simulink model "Import_IMU"  (R2023b)
settings: Solver=FixedStepDiscrete  StartTime=0.0  StopTime=inf  FixedStep=0.003  RelTol=1e-3
InitFcn:
  | run('dual_leg_init.m');
values from neighbouring files (symbols this model uses):
  L1 = single(0.0804)    [dual_leg_init.m]
  L2 = single(0.1200)    [dual_leg_init.m]
  L3 = single(0.1200)    [dual_leg_init.m]
  L4 = single(0.0804)    [dual_leg_init.m]
  L5 = single(0.0700)    [dual_leg_init.m]
undefined symbols (not defined in the file or in its folder): CAL
libraries: ros2lib x14
(part 2 of 2)

== matlab function Import_IMU/FiveBar_IK_Right ==
  data: xCmd input; alphaCmd output; yCmd input; alphaActual input; betaActual input; L1 input; L2 input; L3 input; L4 input; L5 input; betaCmd output; valid output
function [alphaCmd, betaCmd, valid] = fivebar_ik( ...
    xCmd, yCmd, ...
    alphaActual, betaActual, ...
    L1, L2, L3, L4, L5)
%#codegen
%
% Five-Bar Inverse Kinematics
% 五连杆逆运动学
%
% 功能：
% 已知轮毂中心目标坐标(xCmd,yCmd)，
% 求两个主动关节目标角alphaCmd、betaCmd。
%
% 坐标定义：
%
% Alpha电机中心：
%   O = (0,0)
%
% Beta电机中心：
%   D = (L5,0)
%
% 腿部局部坐标：
%   +x：Alpha电机指向Beta电机
%   +y：竖直向下
%
% 连杆：
%   O-A = L1
%   A-B = L2
%   D-C = L4
%   C-B = L3
%
% 输入：
%   xCmd        轮毂目标x，单位m
%   yCmd        轮毂目标y，单位m
%   alphaActual 当前实际Alpha关节角，单位rad
%   betaActual  当前实际Beta关节角，单位rad
%   L1~L5       五连杆尺寸，单位m
%
% 输出：
%   alphaCmd    Alpha关节目标角，单位rad
%   betaCmd     Beta关节目标角，单位rad
%   valid       目标位置是否可达
%
% 解选择方法：
% 每个主动关节都会产生两个候选解，
% 本函数选择最接近当前实际关节角的解，
% 避免机构突然跳到另一种装配构型。

%% 默认输出

alphaCmd = alphaActual;
betaCmd  = betaActual;
valid    = false;

%% 检查输入是否有效

inputValid = ...
    isfinite(xCmd)        && ...
    isfinite(yCmd)        && ...
    isfinite(alphaActual) && ...
    isfinite(betaActual)  && ...
    isfinite(L1)          && ...
    isfinite(L2)          && ...
    isfinite(L3)          && ...
    isfinite(L4)          && ...
    isfinite(L5);

if ~inputValid
    return;
end

if L1 <= single(0) || ...
   L2 <= single(0) || ...
   L3 <= single(0) || ...
   L4 <= single(0) || ...
   L5 <= single(0)

    return;
end

%% =========================================================
%  求Alpha侧两个候选解
%
%  Alpha电机中心O = (0,0)
%  主动杆长度L1
%  被动杆长度L2
% ==========================================================

dxAlpha = xCmd;
dyAlpha = yCmd;

rAlphaSquared = ...
    dxAlpha * dxAlpha + ...
    dyAlpha * dyAlpha;

rAlpha = sqrt(rAlphaSquared);

% 检查目标是否在Alpha侧二连杆工作空间内
if rAlpha < single(1.0e-6)
    return;
end

if rAlpha > L1 + L2
    return;
end

if rAlpha < abs(L1 - L2)
    return;
end

% 从余弦定理求主动杆与目标连线之间的夹角
cosDeltaAlpha = ...
    (L1 * L1 + rAlphaSquared - L2 * L2) / ...
    (single(2) * L1 * rAlpha);

% 处理浮点数误差
tolerance = single(1.0e-5);

if cosDeltaAlpha > single(1) + tolerance || ...
   cosDeltaAlpha < single(-1) - tolerance

    return;
end

if cosDeltaAlpha > single(1)
    cosDeltaAlpha = single(1);
elseif cosDeltaAlpha < single(-1)
    cosDeltaAlpha = single(-1);
end

phiAlpha = atan2(dyAlpha, dxAlpha);
deltaAlpha = acos(cosDeltaAlpha);

% Alpha两个候选角
alphaCandidate1 = phiAlpha + deltaAlpha;
alphaCandidate2 = phiAlpha - deltaAlpha;

%% =========================================================
%  求Beta侧两个候选解
%
%  Beta电机中心D = (L5,0)
%  主动杆长度L4
%  被动杆长度L3
% ==========================================================

dxBeta = xCmd - L5;
dyBeta = yCmd;

rBetaSquared = ...
    dxBeta * dxBeta + ...
    dyBeta * dyBeta;

rBeta = sqrt(rBetaSquared);

% 检查目标是否在Beta侧二连杆工作空间内
if rBeta < single(1.0e-6)
    return;
end

if rBeta > L4 + L3
    return;
end

if rBeta < abs(L4 - L3)
    return;
end

cosDeltaBeta = ...
    (L4 * L4 + rBetaSquared - L3 * L3) / ...
    (single(2) * L4 * rBeta);

if cosDeltaBeta > single(1) + tolerance || ...
   cosDeltaBeta < single(-1) - tolerance

    return;
end

if cosDeltaBeta > single(1)
    cosDeltaBeta = single(1);
elseif cosDeltaBeta < single(-1)
    cosDeltaBeta = single(-1);
end

phiBeta = atan2(dyBeta, dxBeta);
deltaBeta = acos(cosDeltaBeta);

% Beta两个候选角
betaCandidate1 = phiBeta + deltaBeta;
betaCandidate2 = phiBeta - deltaBeta;

%% =========================================================
%  将候选角转换到当前实际关节角附近
%
%  例如：
%  当前角为3.2 rad，
%  候选角为-3.0 rad，
%  实际上二者可能只相差约0.08 rad。
% ==========================================================

alphaCandidate1 = alphaActual + ...
    wrap_to_pi_single(alphaCandidate1 - alphaActual);

alphaCandidate2 = alphaActual + ...
    wrap_to_pi_single(alphaCandidate2 - alphaActual);

betaCandidate1 = betaActual + ...
    wrap_to_pi_single(betaCandidate1 - betaActual);

betaCandidate2 = betaActual + ...
    wrap_to_pi_single(betaCandidate2 - betaActual);

%% 选择距离当前实际角最近的Alpha解

alphaError1 = abs(alphaCandidate1 - alphaActual);
alphaError2 = abs(alphaCandidate2 - alphaActual);

if alphaError1 <= alphaError2
    alphaCmd = alphaCandidate1;
else
    alphaCmd = alphaCandidate2;
end

%% 选择距离当前实际角最近的Beta解

betaError1 = abs(betaCandidate1 - betaActual);
betaError2 = abs(betaCandidate2 - betaActual);

if betaError1 <= betaError2
    betaCmd = betaCandidate1;
else
    betaCmd = betaCandidate2;
end

%% 最终有效性检查

if ~isfinite(alphaCmd) || ~isfinite(betaCmd)
    alphaCmd = alphaActual;
    betaCmd  = betaActual;
    return;
end

valid = true;

end


function angleWrapped = wrap_to_pi_single(angle)
% 将角度限制到[-pi,pi)

piSingle = single(pi);
twoPi = single(2) * piSingle;

angleWrapped = mod(angle + piSingle, twoPi) - piSingle;

end

== matlab function Import_IMU/Right_leg/Right_Joint_To_Motor_R ==
  data: alpha_cmd input; p_RA_target output; beta_cmd input; p_RB_target output; valid output
function [p_RA_target, p_RB_target, valid] = ...
    Right_Joint_To_Motor(alpha_cmd, beta_cmd)
%#codegen
% 将左腿两个主动关节目标角转换为电机目标角

% RA标定参数
qm0_RA   = single(-0.9126806259155273);
qj0_RA   = single(2.2416795698181398);
sign_RA  = single( 1.0);
ratio_RA = single( 1.0);

% RB标定参数
qm0_RB   = single(-0.6025409698486328);
qj0_RB   = single(-0.36295295726680576);
sign_RB  = single( 1.0);
ratio_RB = single( 1.0);

alpha_cmd = single(alpha_cmd);
beta_cmd  = single(beta_cmd);

p_RA_target = qm0_RA + ...
    (alpha_cmd - qj0_RA) * ratio_RA / sign_RA;

p_RB_target = qm0_RB + ...
    (beta_cmd - qj0_RB) * ratio_RB / sign_RB;

valid = ...
    isfinite(p_RA_target) && ...
    isfinite(p_RB_target);

end

== matlab function Import_IMU/Right_leg/Motor_Target_Velocity_LA ==
  data: p_cmd input; v_des output; enable input; Ts input; cutoff_hz input; max_velocity input; valid output
function [v_des, valid] = Motor_Target_Velocity( ...
    p_cmd, enable, Ts, cutoff_hz, max_velocity)
%#codegen
% 根据最终电机位置目标计算速度目标
%
% p_cmd        最终发送的电机目标位置，rad
% enable       控制使能
% Ts           控制周期，s
% cutoff_hz    速度低通滤波截止频率，Hz
% max_velocity 目标速度限制，rad/s

persistent p_previous
persistent v_previous
persistent was_enabled

if isempty(p_previous)
    p_previous = single(0);
    v_previous = single(0);
    was_enabled = false;
end

p_cmd        = single(p_cmd);
Ts           = single(Ts);
cutoff_hz    = single(cutoff_hz);
max_velocity = single(max_velocity);

v_des = single(0);
valid = false;

control_enabled = enable ~= 0;

if ~control_enabled
    p_previous = p_cmd;
    v_previous = single(0);
    was_enabled = false;
    return;
end

if ~isfinite(p_cmd) || ...
   ~isfinite(Ts) || ...
   ~isfinite(cutoff_hz) || ...
   ~isfinite(max_velocity)
    return;
end

if Ts <= single(1.0e-6)
    return;
end

% 刚使能时避免产生巨大差分速度
if ~was_enabled
    p_previous = p_cmd;
    v_previous = single(0);
    was_enabled = true;

    v_des = single(0);
    valid = true;
    return;
end

% 原始差分速度
v_raw = (p_cmd - p_previous) / Ts;

% 速度限幅
v_raw = min(max(v_raw, -max_velocity), max_velocity);

% 一阶低通滤波
if cutoff_hz > single(0)
    filter_coefficient = ...
        exp(-single(2.0*pi) * cutoff_hz * Ts);

    v_des = ...
        filter_coefficient * v_previous + ...
        (single(1.0) - filter_coefficient) * v_raw;
else
    v_des = v_raw;
end

% 再做一次限幅
v_des = min(max(v_des, -max_velocity), max_velocity);

p_previous = p_cmd;
v_previous = v_des;

valid = isfinite(v_des);

end

== matlab function Import_IMU/Right_leg/Motor_Target_Velocity_LB ==
  data: p_cmd input; v_des output; enable input; Ts input; cutoff_hz input; max_velocity input; valid output
function [v_des, valid] = Motor_Target_Velocity( ...
    p_cmd, enable, Ts, cutoff_hz, max_velocity)
%#codegen
% 根据最终电机位置目标计算速度目标
%
% p_cmd        最终发送的电机目标位置，rad
% enable       控制使能
% Ts           控制周期，s
% cutoff_hz    速度低通滤波截止频率，Hz
% max_velocity 目标速度限制，rad/s

persistent p_previous
persistent v_previous
persistent was_enabled

if isempty(p_previous)
    p_previous = single(0);
    v_previous = single(0);
    was_enabled = false;
end

p_cmd        = single(p_cmd);
Ts           = single(Ts);
cutoff_hz    = single(cutoff_hz);
max_velocity = single(max_velocity);

v_des = single(0);
valid = false;

control_enabled = enable ~= 0;

if ~control_enabled
    p_previous = p_cmd;
    v_previous = single(0);
    was_enabled = false;
    return;
end

if ~isfinite(p_cmd) || ...
   ~isfinite(Ts) || ...
   ~isfinite(cutoff_hz) || ...
   ~isfinite(max_velocity)
    return;
end

if Ts <= single(1.0e-6)
    return;
end

% 刚使能时避免产生巨大差分速度
if ~was_enabled
    p_previous = p_cmd;
    v_previous = single(0);
    was_enabled = true;

    v_des = single(0);
    valid = true;
    return;
end

% 原始差分速度
v_raw = (p_cmd - p_previous) / Ts;

% 速度限幅
v_raw = min(max(v_raw, -max_velocity), max_velocity);

% 一阶低通滤波
if cutoff_hz > single(0)
    filter_coefficient = ...
        exp(-single(2.0*pi) * cutoff_hz * Ts);

    v_des = ...
        filter_coefficient * v_previous + ...
        (single(1.0) - filter_coefficient) * v_raw;
else
    v_des = v_raw;
end

% 再做一次限幅
v_des = min(max(v_des, -max_velocity), max_velocity);

p_previous = p_cmd;
v_previous = v_des;

valid = isfinite(v_des);

end

== matlab function Import_IMU/Switch/RC_Safety_Gate ==
  data: isNew input; enable_safe output; online input; rightSwitch input; rc_alive output; rc_ready output; status output
function [enable_safe,rc_alive,rc_ready,status] = ...
    RC_Safety_Gate(isNew,online,rightSwitch)
%#codegen
%
% isNew       : ROS 2 Subscribe的IsNew端口，boolean
% online      : ReadDJIRC.online，uint8
% rightSwitch : ReadDJIRC.right_switch，uint8
%
% enable_safe : 最终安全使能
% rc_alive    : 遥控器通信正常
% rc_ready    : 已经先经过失能挡，可以允许使能
% status      : 状态码，方便调试

persistent missedCount receivedOnce seenDisable

if isempty(missedCount)
    % 启动时直接处于超时状态
    missedCount = uint32(34);
    receivedOnce = false;
    seenDisable = false;
end

% 当前模型Ts = 0.003 s
% 0.1 / 0.003 = 33.33
% 所以连续34个周期没有新消息就判定超时
TIMEOUT_STEPS = uint32(34);

%% 1. 新消息计数与超时判断
if isNew
    missedCount = uint32(0);
    receivedOnce = true;
else
    if missedCount < uint32(1000000)
        missedCount = missedCount + uint32(1);
    end
end

fresh = receivedOnce && ...
        (missedCount < TIMEOUT_STEPS);

%% 2. 检查遥控器消息是否合法
% 你的右侧三档开关正常值应为1、2、3
switchValid = ...
    (rightSwitch >= uint8(1)) && ...
    (rightSwitch <= uint8(3));

rc_alive = fresh && ...
           (online ~= uint8(0)) && ...
           switchValid;

%% 3. 启动互锁
% 一旦断线，清除“见过失能挡”的记录。
% 这样重新连接时，即使开关仍在3挡，也不会自动使能。
if ~rc_alive
    seenDisable = false;
else
    % 当前模型中 right_switch > 2 才使能，
    % 因此1挡和2挡都看作失能状态。
    if rightSwitch <= uint8(2)
        seenDisable = true;
    end
end

rc_ready = rc_alive && seenDisable;

%% 4. 最终使能
% 必须：
% 通信正常
% 已经先经过失能挡
% 当前开关位于3挡
enable_safe = rc_ready && ...
              (rightSwitch == uint8(3));

%% 5. 状态码
% 0：从未收到消息
% 1：消息超时
% 2：online=0或开关值非法
% 3：等待先拨到失能挡
% 4：通信正常，当前处于失能挡
% 5：安全使能
status = uint8(0);

if ~receivedOnce
    status = uint8(0);
elseif ~fresh
    status = uint8(1);
elseif (online == uint8(0)) || ~switchValid
    status = uint8(2);
elseif ~seenDisable
    status = uint8(3);
elseif rightSwitch <= uint8(2)
    status = uint8(4);
else
    status = uint8(5);
end
end

== matlab function Import_IMU/Wheel_Pitch_Controller ==
  data: enableSafe input; wheelEnable output; imuValid input; pitch input; gyroY input; wheelVelocityLeft input; wheelVelocityRight input; KpVelocity input; KpPitch input; KdPitch input; torqueLimit input; tauCommon output; pitchCmd output; pitchError output; wheelVelocityAverage output
function [wheelEnable,tauCommon,pitchCmd,pitchError,wheelVelocityAverage] = ...
    Wheel_Pitch_Controller( ...
    enableSafe,imuValid, ...
    pitch,gyroY, ...
    wheelVelocityLeft,wheelVelocityRight, ...
    KpVelocity,KpPitch,KdPitch,torqueLimit)
%#codegen
%
% 轮腿机器人精简Pitch平衡控制器
%
% 控制结构：
%   轮速外环 P -> pitchCmd
%   Pitch内环 PD -> tauCommon
%
% switch=3使enableSafe变为1时：
%   关节开始回腿
%   轮毂平衡同时立即启动
%
% 单位：
%   pitch               rad
%   gyroY               rad/s
%   wheelVelocity       rad/s
%
% 左右轮安装方向在模块外部通过Gain处理。

persistent torqueBlend
persistent wasEnabled

if isempty(torqueBlend)
    torqueBlend = single(0);
    wasEnabled = false;
end

%% 固定参数

Ts = single(0.003);

% 轮毂闭环立即启动，但力矩在0.2秒内平滑增加
softStartTime = single(0.2);

% 速度外环生成的Pitch目标最大为±3度
pitchCmdLimit = single(0.05236);

% Pitch超过20度时停止轮毂使能
fallAngleLimit = single(0.34907);

%% 默认输出

wheelEnable = false;

tauCommon = single(0);
pitchCmd = single(0);
pitchError = single(0);
wheelVelocityAverage = single(0);

%% 最小有效性判断

dataValid = ...
    logical(imuValid) && ...
    isfinite(pitch) && ...
    isfinite(gyroY) && ...
    isfinite(wheelVelocityLeft) && ...
    isfinite(wheelVelocityRight) && ...
    isfinite(KpVelocity) && ...
    isfinite(KpPitch) && ...
    isfinite(KdPitch) && ...
    isfinite(torqueLimit) && ...
    torqueLimit >= single(0);

angleSafe = abs(pitch) < fallAngleLimit;

wheelEnable = ...
    logical(enableSafe) && ...
    dataValid && ...
    angleSafe;

%% 失能时复位

if ~wheelEnable

    torqueBlend = single(0);
    wasEnabled = false;

    return;
end

%% 使能上升沿

if ~wasEnabled
    torqueBlend = single(0);
end

wasEnabled = true;

%% 左右平均轮速

% 前提：
% 左右轮速度已经在模块外通过Gain统一为：
% 机器人向前运动时都为正。

wheelVelocityAverage = ...
    single(0.5) * ...
    (wheelVelocityLeft + wheelVelocityRight);

%% 速度外环

% 当前目标速度固定为0。
% 机器人向前滚时，速度误差为负。

velocityCmd = single(0);
velocityError = velocityCmd - wheelVelocityAverage;

pitchCmdRaw = KpVelocity * velocityError;

if pitchCmdRaw > pitchCmdLimit
    pitchCmd = pitchCmdLimit;
elseif pitchCmdRaw < -pitchCmdLimit
    pitchCmd = -pitchCmdLimit;
else
    pitchCmd = pitchCmdRaw;
end

%% Pitch姿态内环

pitchError = pitchCmd - pitch;

% 假设：
% gyroY为正时，Pitch正在向正方向增大。
%
% P项把Pitch拉回目标。
% D项抑制Pitch角速度。

tauRaw = ...
    KpPitch * pitchError ...
    - KdPitch * gyroY;

%% 力矩限幅

if tauRaw > torqueLimit
    tauCommon = torqueLimit;
elseif tauRaw < -torqueLimit
    tauCommon = -torqueLimit;
else
    tauCommon = tauRaw;
end

%% 力矩软启动

% 闭环在enableSafe上升沿立即运行，
% 仅将实际输出力矩平滑增加，防止第一帧突变。

if softStartTime <= Ts

    torqueBlend = single(1);

else

    torqueBlend = ...
        torqueBlend + Ts / softStartTime;

    if torqueBlend > single(1)
        torqueBlend = single(1);
    end
end

tauCommon = tauCommon * torqueBlend;

end

== matlab function Import_IMU/Motor_To_Joint_LA/Motor_Position_To_Joint ==
  data: q_motor input; q_joint output; q_motor_ref input; q_joint_ref input; motor_sign input; motor_ratio input
function q_joint = motor_position_to_joint( ...
    q_motor, q_motor_ref, q_joint_ref, ...
    motor_sign, motor_ratio)
%#codegen
%
% 电机编码器位置转换为运动学关节角
%
% q_motor      当前电机位置
% q_motor_ref  标定姿态下电机位置
% q_joint_ref  标定姿态下理论关节角
% motor_sign   方向修正：+1或-1
% motor_ratio  传动比

q_joint = q_joint_ref;

if abs(motor_ratio) > single(1.0e-6)
    q_joint = ...
        (q_motor - q_motor_ref) ...
        * motor_sign / motor_ratio ...
        + q_joint_ref;
end
end

== matlab function Import_IMU/Yaw_Hold_Controller ==
  data: enableSafe input; tauYaw output; wheelEnable input; imuValid input; yaw input; gyroZ input; KpYaw input; KdYaw input; YawTorqueLimit input; yawTarget output; yawError output; yawHoldActive output
function [tauYaw,yawTarget,yawError,yawHoldActive] = ...
    Yaw_Hold_Controller( ...
    enableSafe,wheelEnable,imuValid, ...
    yaw,gyroZ, ...
    KpYaw,KdYaw,YawTorqueLimit)
%#codegen

persistent yawReference
persistent previousCaptureEnable

if isempty(yawReference)
    yawReference = single(0);
    previousCaptureEnable = false;
end

%% 常量
piValue = single(3.141592653589793);
twoPi = single(6.283185307179586);

% 避免零点附近因IMU噪声反复修正
yawDeadband = single(0.00872665);  % 约0.5°
gyroDeadband = single(0.02);      % rad/s

%% 默认输出
tauYaw = single(0);
yawTarget = yawReference;
yawError = single(0);
yawHoldActive = false;

%% 检查信号
yawValid = ...
    logical(imuValid) && ...
    isfinite(yaw);

captureEnable = ...
    logical(enableSafe) && ...
    yawValid;

%% 右开关从非3档进入3档时，锁定当前Yaw
if captureEnable && ~previousCaptureEnable
    yawReference = yaw;
end

previousCaptureEnable = captureEnable;
yawTarget = yawReference;

%% 控制有效性
controlValid = ...
    captureEnable && ...
    logical(wheelEnable) && ...
    isfinite(gyroZ) && ...
    isfinite(KpYaw) && ...
    isfinite(KdYaw) && ...
    isfinite(YawTorqueLimit) && ...
    KpYaw >= single(0) && ...
    KdYaw >= single(0) && ...
    YawTorqueLimit >= single(0);

if ~controlValid
    tauYaw = single(0);
    return;
end

yawHoldActive = true;

%% Yaw误差
yawError = yawReference - yaw;

% 将误差限制到[-pi, pi]
while yawError > piValue
    yawError = yawError - twoPi;
end

while yawError < -piValue
    yawError = yawError + twoPi;
end

%% Yaw角误差平滑死区
if yawError > yawDeadband
    yawErrorEffective = yawError - yawDeadband;

elseif yawError < -yawDeadband
    yawErrorEffective = yawError + yawDeadband;

else
    yawErrorEffective = single(0);
end

%% GyroZ平滑死区
if gyroZ > gyroDeadband
    gyroZEffective = gyroZ - gyroDeadband;

elseif gyroZ < -gyroDeadband
    gyroZEffective = gyroZ + gyroDeadband;

else
    gyroZEffective = single(0);
end

%% Yaw PD控制
tauYawRaw = ...
    KpYaw * yawErrorEffective ...
    - KdYaw * gyroZEffective;

%% Yaw力矩限幅
if tauYawRaw > YawTorqueLimit
    tauYaw = YawTorqueLimit;

elseif tauYawRaw < -YawTorqueLimit
    tauYaw = -YawTorqueLimit;

else
    tauYaw = tauYawRaw;
end

end

== matlab function Import_IMU/Left_leg/Left_Joint_To_Motor_L ==
  data: alpha_cmd input; p_LA_target output; beta_cmd input; p_LB_target output; valid output
function [p_LA_target, p_LB_target, valid] = ...
    Left_Joint_To_Motor(alpha_cmd, beta_cmd)
%#codegen
% 将左腿两个主动关节目标角转换为电机目标角

% LA标定参数
qm0_LA   = single(-0.3408479690551758);
qj0_LA   = single( 3.504545610856599);
sign_LA  = single(-1.0);
ratio_LA = single( 1.0);

% LB标定参数
qm0_LB   = single(-0.6292438507080078);
qj0_LB   = single( 0.8999130837716534);
sign_LB  = single(-1.0);
ratio_LB = single( 1.0);

alpha_cmd = single(alpha_cmd);
beta_cmd  = single(beta_cmd);

p_LA_target = qm0_LA + ...
    (alpha_cmd - qj0_LA) * ratio_LA / sign_LA;

p_LB_target = qm0_LB + ...
    (beta_cmd - qj0_LB) * ratio_LB / sign_LB;

valid = ...
    isfinite(p_LA_target) && ...
    isfinite(p_LB_target);

end

== matlab function Import_IMU/Left_leg/Motor_Target_Velocity_LA ==
  data: p_cmd input; v_des output; enable input; Ts input; cutoff_hz input; max_velocity input; valid output
function [v_des, valid] = Motor_Target_Velocity( ...
    p_cmd, enable, Ts, cutoff_hz, max_velocity)
%#codegen
% 根据最终电机位置目标计算速度目标
%
% p_cmd        最终发送的电机目标位置，rad
% enable       控制使能
% Ts           控制周期，s
% cutoff_hz    速度低通滤波截止频率，Hz
% max_velocity 目标速度限制，rad/s

persistent p_previous
persistent v_previous
persistent was_enabled

if isempty(p_previous)
    p_previous = single(0);
    v_previous = single(0);
    was_enabled = false;
end

p_cmd        = single(p_cmd);
Ts           = single(Ts);
cutoff_hz    = single(cutoff_hz);
max_velocity = single(max_velocity);

v_des = single(0);
valid = false;

control_enabled = enable ~= 0;

if ~control_enabled
    p_previous = p_cmd;
    v_previous = single(0);
    was_enabled = false;
    return;
end

if ~isfinite(p_cmd) || ...
   ~isfinite(Ts) || ...
   ~isfinite(cutoff_hz) || ...
   ~isfinite(max_velocity)
    return;
end

if Ts <= single(1.0e-6)
    return;
end

% 刚使能时避免产生巨大差分速度
if ~was_enabled
    p_previous = p_cmd;
    v_previous = single(0);
    was_enabled = true;

    v_des = single(0);
    valid = true;
    return;
end

% 原始差分速度
v_raw = (p_cmd - p_previous) / Ts;

% 速度限幅
v_raw = min(max(v_raw, -max_velocity), max_velocity);

% 一阶低通滤波
if cutoff_hz > single(0)
    filter_coefficient = ...
        exp(-single(2.0*pi) * cutoff_hz * Ts);

    v_des = ...
        filter_coefficient * v_previous + ...
        (single(1.0) - filter_coefficient) * v_raw;
else
    v_des = v_raw;
end

% 再做一次限幅
v_des = min(max(v_des, -max_velocity), max_velocity);

p_previous = p_cmd;
v_previous = v_des;

valid = isfinite(v_des);

end

== matlab function Import_IMU/Left_leg/Motor_Target_Velocity_LB ==
  data: p_cmd input; v_des output; enable input; Ts input; cutoff_hz input; max_velocity input; valid output
function [v_des, valid] = Motor_Target_Velocity( ...
    p_cmd, enable, Ts, cutoff_hz, max_velocity)
%#codegen
% 根据最终电机位置目标计算速度目标
%
% p_cmd        最终发送的电机目标位置，rad
% enable       控制使能
% Ts           控制周期，s
% cutoff_hz    速度低通滤波截止频率，Hz
% max_velocity 目标速度限制，rad/s

persistent p_previous
persistent v_previous
persistent was_enabled

if isempty(p_previous)
    p_previous = single(0);
    v_previous = single(0);
    was_enabled = false;
end

p_cmd        = single(p_cmd);
Ts           = single(Ts);
cutoff_hz    = single(cutoff_hz);
max_velocity = single(max_velocity);

v_des = single(0);
valid = false;

control_enabled = enable ~= 0;

if ~control_enabled
    p_previous = p_cmd;
    v_previous = single(0);
    was_enabled = false;
    return;
end

if ~isfinite(p_cmd) || ...
   ~isfinite(Ts) || ...
   ~isfinite(cutoff_hz) || ...
   ~isfinite(max_velocity)
    return;
end

if Ts <= single(1.0e-6)
    return;
end

% 刚使能时避免产生巨大差分速度
if ~was_enabled
    p_previous = p_cmd;
    v_previous = single(0);
    was_enabled = true;

    v_des = single(0);
    valid = true;
    return;
end

% 原始差分速度
v_raw = (p_cmd - p_previous) / Ts;

% 速度限幅
v_raw = min(max(v_raw, -max_velocity), max_velocity);

% 一阶低通滤波
if cutoff_hz > single(0)
    filter_coefficient = ...
        exp(-single(2.0*pi) * cutoff_hz * Ts);

    v_des = ...
        filter_coefficient * v_previous + ...
        (single(1.0) - filter_coefficient) * v_raw;
else
    v_des = v_raw;
end

% 再做一次限幅
v_des = min(max(v_des, -max_velocity), max_velocity);

p_previous = p_cmd;
v_previous = v_des;

valid = isfinite(v_des);

end

== matlab function Import_IMU/Wheel_Torque_Mixer ==
  data: tauPitch input; tauLeftPhysical output; tauYawRequest input; TotalTorqueLimit input; YawDirection input; tauRightPhysical output; tauYawUsed output
function [tauLeftPhysical,tauRightPhysical,tauYawUsed] = ...
    Wheel_Torque_Mixer( ...
    tauPitch,tauYawRequest, ...
    TotalTorqueLimit,YawDirection)
%#codegen

%% 默认输出
tauLeftPhysical = single(0);
tauRightPhysical = single(0);
tauYawUsed = single(0);

%% 输入检查
if ~isfinite(tauPitch) || ...
   ~isfinite(tauYawRequest) || ...
   ~isfinite(TotalTorqueLimit) || ...
   ~isfinite(YawDirection) || ...
   TotalTorqueLimit < single(0)
    return;
end

%% Pitch公共力矩先限幅
if tauPitch > TotalTorqueLimit
    tauPitchLimited = TotalTorqueLimit;

elseif tauPitch < -TotalTorqueLimit
    tauPitchLimited = -TotalTorqueLimit;

else
    tauPitchLimited = tauPitch;
end

%% Yaw方向修正
tauYawSigned = YawDirection * tauYawRequest;

%% 优先保证Pitch平衡
% 例如总限幅0.1，Pitch已经使用0.08，
% 那么Yaw最多只能再使用0.02。
yawHeadroom = ...
    TotalTorqueLimit - abs(tauPitchLimited);

if yawHeadroom < single(0)
    yawHeadroom = single(0);
end

%% 限制实际Yaw力矩
if tauYawSigned > yawHeadroom
    tauYawUsed = yawHeadroom;

elseif tauYawSigned < -yawHeadroom
    tauYawUsed = -yawHeadroom;

else
    tauYawUsed = tauYawSigned;
end

%% 公共Pitch力矩 + 差动Yaw力矩
tauLeftPhysical = ...
    tauPitchLimited - tauYawUsed;

tauRightPhysical = ...
    tauPitchLimited + tauYawUsed;

end

== matlab function Import_IMU/RC setting/PWM ==
  data: u input; y output
function y = fcn(u)
y = u*500+1500;

== matlab function Import_IMU/RC setting/PWM1 ==
  data: u input; y output
function y = fcn(u)
y = u*500+1500;

== matlab function Import_IMU/RC setting/PWM2 ==
  data: u input; y output
function y = fcn(u)
y = u*500+1500;

== matlab function Import_IMU/RC setting/Deadzone ==
  data: u input; y output
function y = fcn(u)
%#codegen
% 输入范围约为 [-1, 1]
% 输出范围为 [-1, 1]
% 中心死区为 ±0.05

u = single(u);

deadZone = single(0.05);
oneValue = single(1.0);
zeroValue = single(0.0);

% 先限制输入范围
if u > oneValue
    u = oneValue;
elseif u < -oneValue
    u = -oneValue;
end

% 死区处理，并重新映射，使死区外仍覆盖 [-1,1]
if u > deadZone
    y = (u - deadZone) / (oneValue - deadZone);
elseif u < -deadZone
    y = (u + deadZone) / (oneValue - deadZone);
else
    y = zeroValue;
end

end

== matlab function Import_IMU/RC setting/Deadzone1 ==
  data: u input; y output
function y = fcn(u)
%#codegen
% 输入范围约为 [-1, 1]
% 输出范围为 [-1, 1]
% 中心死区为 ±0.05

u = single(u);

deadZone = single(0.05);
oneValue = single(1.0);
zeroValue = single(0.0);

% 先限制输入范围
if u > oneValue
    u = oneValue;
elseif u < -oneValue
    u = -oneValue;
end

% 死区处理，并重新映射，使死区外仍覆盖 [-1,1]
if u > deadZone
    y = (u - deadZone) / (oneValue - deadZone);
elseif u < -deadZone
    y = (u + deadZone) / (oneValue - deadZone);
else
    y = zeroValue;
end

end

== matlab function Import_IMU/RC setting/Deadzone2 ==
  data: u input; y output
function y = fcn(u)
%#codegen
% 输入范围约为 [-1, 1]
% 输出范围为 [-1, 1]
% 中心死区为 ±0.05

u = single(u);

deadZone = single(0.05);
oneValue = single(1.0);
zeroValue = single(0.0);

% 先限制输入范围
if u > oneValue
    u = oneValue;
elseif u < -oneValue
    u = -oneValue;
end

% 死区处理，并重新映射，使死区外仍覆盖 [-1,1]
if u > deadZone
    y = (u - deadZone) / (oneValue - deadZone);
elseif u < -deadZone
    y = (u + deadZone) / (oneValue - deadZone);
else
    y = zeroValue;
end

end

== matlab function Import_IMU/Motor_Position_To_Joint ==
  data: q_motor input; q_joint output; q_motor_ref input; q_joint_ref input; motor_sign input; motor_ratio input
function q_joint = motor_position_to_joint( ...
    q_motor, q_motor_ref, q_joint_ref, ...
    motor_sign, motor_ratio)
%#codegen
%
% 电机编码器位置转换为运动学关节角
%
% q_motor      当前电机位置
% q_motor_ref  标定姿态下电机位置
% q_joint_ref  标定姿态下理论关节角
% motor_sign   方向修正：+1或-1
% motor_ratio  传动比

q_joint = q_joint_ref;

if abs(motor_ratio) > single(1.0e-6)
    q_joint = ...
        (q_motor - q_motor_ref) ...
        * motor_sign / motor_ratio ...
        + q_joint_ref;
end
end

== matlab function Import_IMU/Motor_To_Joint_LB/Motor_Position_To_Joint ==
  data: q_motor input; q_joint output; q_motor_ref input; q_joint_ref input; motor_sign input; motor_ratio input
function q_joint = motor_position_to_joint( ...
    q_motor, q_motor_ref, q_joint_ref, ...
    motor_sign, motor_ratio)
%#codegen
%
% 电机编码器位置转换为运动学关节角
%
% q_motor      当前电机位置
% q_motor_ref  标定姿态下电机位置
% q_joint_ref  标定姿态下理论关节角
% motor_sign   方向修正：+1或-1
% motor_ratio  传动比

q_joint = q_joint_ref;

if abs(motor_ratio) > single(1.0e-6)
    q_joint = ...
        (q_motor - q_motor_ref) ...
        * motor_sign / motor_ratio ...
        + q_joint_ref;
end
end

== matlab function Import_IMU/Motor_To_Joint_RA/Motor_Position_To_Joint ==
  data: q_motor input; q_joint output; q_motor_ref input; q_joint_ref input; motor_sign input; motor_ratio input
function q_joint = motor_position_to_joint( ...
    q_motor, q_motor_ref, q_joint_ref, ...
    motor_sign, motor_ratio)
%#codegen
%
% 电机编码器位置转换为运动学关节角
%
% q_motor      当前电机位置
% q_motor_ref  标定姿态下电机位置
% q_joint_ref  标定姿态下理论关节角
% motor_sign   方向修正：+1或-1
% motor_ratio  传动比

q_joint = q_joint_ref;

if abs(motor_ratio) > single(1.0e-6)
    q_joint = ...
        (q_motor - q_motor_ref) ...
        * motor_sign / motor_ratio ...
        + q_joint_ref;
end
end

== matlab function Import_IMU/Motor_To_Joint_RB/Motor_Position_To_Joint ==
  data: q_motor input; q_joint output; q_motor_ref input; q_joint_ref input; motor_sign input; motor_ratio input
function q_joint = motor_position_to_joint( ...
    q_motor, q_motor_ref, q_joint_ref, ...
    motor_sign, motor_ratio)
%#codegen
%
% 电机编码器位置转换为运动学关节角
%
% q_motor      当前电机位置
% q_motor_ref  标定姿态下电机位置
% q_joint_ref  标定姿态下理论关节角
% motor_sign   方向修正：+1或-1
% motor_ratio  传动比

q_joint = q_joint_ref;

if abs(motor_ratio) > single(1.0e-6)
    q_joint = ...
        (q_motor - q_motor_ref) ...
        * motor_sign / motor_ratio ...
        + q_joint_ref;
end
end

== matlab function Import_IMU/FiveBar_FK_Left ==
  data: alpha input; xB output; beta input; L1 input; L2 input; L3 input; L4 input; L5 input; yB output; leg_length output; leg_angle output; valid output
function [xB, yB, leg_length, leg_angle, valid] = ...
    fivebar_fk_actual(alpha, beta, L1, L2, L3, L4, L5)
%#codegen
%
% 五连杆正运动学
%
% 坐标定义：
% O = (0,0)
% D = (L5,0)
% +x：Alpha电机指向Beta电机
% +y：竖直向下
%
% alpha：O点主动杆角度
% beta ：D点主动杆角度
%
% 输出：
% xB、yB       轮心坐标
% leg_length   基座中点到轮心的虚拟腿长
% leg_angle    虚拟腿相对竖直向下方向的角度
% valid        正运动学是否有效

xB = single(0);
yB = single(0);
leg_length = single(0);
leg_angle = single(0);
valid = false;

%% 主动杆末端A
Ax = L1 * cos(alpha);
Ay = L1 * sin(alpha);

%% 主动杆末端C
Cx = L5 + L4 * cos(beta);
Cy = L4 * sin(beta);

%% A到C的向量
dx = Cx - Ax;
dy = Cy - Ay;

Dac = sqrt(dx*dx + dy*dy);

%% 可达性检查
if Dac < single(1.0e-6)
    return;
end

if Dac > L2 + L3
    return;
end

if Dac < abs(L2 - L3)
    return;
end

%% 两圆交点
a = (L2*L2 - L3*L3 + Dac*Dac) / ...
    (single(2.0) * Dac);

h2 = L2*L2 - a*a;

if h2 < single(-1.0e-7)
    return;
end

if h2 < single(0)
    h2 = single(0);
end

h = sqrt(h2);

ux = dx / Dac;
uy = dy / Dac;

Mx = Ax + a * ux;
My = Ay + a * uy;

%% 两个候选轮心位置
x1 = Mx - h * uy;
y1 = My + h * ux;

x2 = Mx + h * uy;
y2 = My - h * ux;

%% 当前机构中轮心位于更下方，选择y较大的交点
if y1 >= y2
    xB = x1;
    yB = y1;
else
    xB = x2;
    yB = y2;
end

%% 虚拟腿状态
xMid = xB - L5 / single(2.0);

leg_length = sqrt(xMid*xMid + yB*yB);

% 相对于竖直向下方向
leg_angle = atan2(xMid, yB);

valid = true;
end
